simulink model "Torque_System_Identification"  (R2018a)
settings: Solver=FixedStepAuto  StartTime=0.0  StopTime=inf  FixedStep=.015  RelTol=1e-3  EnableMultiTasking=on
libraries: raspberrypilib x28, hdlsllib x25, simulink x15
(part 2 of 2)

== system Torque_System_Identification/Control System/Black Box/radio_steering read message (Master --> Slave) ==
  Inport : Inport
  Mux : Mux
      settings: DisplayOption=signals
  Read Bit Set : simulink/Logic and Bit Operations/Bit Set  iBit=7
      settings: SourceProductName=Simulink  SourceProductBaseCode=SL
  uint8_t 1 : Constant  OutDataTypeStr=uint8
  uint8_t 2 : Constant  OutDataTypeStr=uint8
  uint8_t 3 : Constant  OutDataTypeStr=uint8
  Out1 : Outport
  wires:
  Read Bit Set/1 -> Mux/1  "Addres/RW Byte radio_steering Teensy Status will be returned here"
  uint8_t 1/1 -> Mux/2  "Junk will be returned here"
  Inport/1 -> Read Bit Set/1
  uint8_t 3/1 -> Mux/4  "Byte 1 will be returned here"
  Mux/1 -> Out1/1
  uint8_t 2/1 -> Mux/3  "Byte 0 will be returned here"

== system Torque_System_Identification/Control System/Black Box/radio_steering return message (Slave --> Master) ==
  In1 : Inport
  8 bytes concatinated converted to double : DataTypeConversion  OutDataTypeStr=double  RndMeth=Nearest
  Bit Concat : hdlsllib/Logic and Bit Operations/Bit Concat  numInputs=2
      settings: SourceProductName=HDL Coder  SourceProductBaseCode=HD
  Bytes of the return message : Display
      settings: Format=decimal (Stored Integer)
  Data Type Conversion : DataTypeConversion  OutDataTypeStr=int16  RndMeth=Nearest
  Demux : Demux
  Display : Display
      settings: Format=binary (Stored Integer)
  Display1 : Display
      settings: Format=decimal (Stored Integer)
  Display2 : Display
      settings: Format=binary (Stored Integer)
  radio_steering : Outport
  wires:
  8 bytes concatinated converted to double/1 -> Display1/1, radio_steering/1  "radio_steering"
  Demux/2 -> Display2/1  "Slave Status"
  Demux/1 -> Display/1  "Previous Data"
  In1/1 -> Bytes of the return message/1, Demux/1
  Bit Concat/1 -> Data Type Conversion/1
  Demux/4 -> Bit Concat/1
  Demux/3 -> Bit Concat/2
  Data Type Conversion/1 -> 8 bytes concatinated converted to double/1

== system Torque_System_Identification/Control System/Black Box/radio_throttle read message (Master --> Slave) ==
  Inport : Inport
  Mux : Mux
      settings: DisplayOption=signals
  Read Bit Set : simulink/Logic and Bit Operations/Bit Set  iBit=7
      settings: SourceProductName=Simulink  SourceProductBaseCode=SL
  uint8_t 1 : Constant  OutDataTypeStr=uint8
  uint8_t 2 : Constant  OutDataTypeStr=uint8
  uint8_t 3 : Constant  OutDataTypeStr=uint8
  Out1 : Outport
  wires:
  Read Bit Set/1 -> Mux/1  "Addres/RW Byte radio_throttle Teensy Status will be returned here"
  uint8_t 1/1 -> Mux/2  "Junk will be returned here"
  Inport/1 -> Read Bit Set/1
  uint8_t 3/1 -> Mux/4  "Byte 1 will be returned here"
  Mux/1 -> Out1/1
  uint8_t 2/1 -> Mux/3  "Byte 0 will be returned here"

== system Torque_System_Identification/Control System/Black Box/radio_throttle return message (Slave --> Master) ==
  In1 : Inport
  8 bytes concatinated converted to double : DataTypeConversion  OutDataTypeStr=double  RndMeth=Nearest
  Bit Concat : hdlsllib/Logic and Bit Operations/Bit Concat  numInputs=2
      settings: SourceProductName=HDL Coder  SourceProductBaseCode=HD
  Bytes of the return message : Display
      settings: Format=decimal (Stored Integer)
  Data Type Conversion : DataTypeConversion  OutDataTypeStr=int16  RndMeth=Nearest
  Demux : Demux
  Display : Display
      settings: Format=binary (Stored Integer)
  Display1 : Display
      settings: Format=decimal (Stored Integer)
  Display2 : Display
      settings: Format=binary (Stored Integer)
  radio_throttle : Outport
  wires:
  8 bytes concatinated converted to double/1 -> Display1/1, radio_throttle/1  "radio_throttle"
  Demux/2 -> Display2/1  "Slave Status"
  Demux/1 -> Display/1  "Previous Data"
  In1/1 -> Bytes of the return message/1, Demux/1
  Bit Concat/1 -> Data Type Conversion/1
  Demux/4 -> Bit Concat/1
  Demux/3 -> Bit Concat/2
  Data Type Conversion/1 -> 8 bytes concatinated converted to double/1

== system Torque_System_Identification/Control System/Black Box/servo_out Write Message (Master --> Slave) ==
  In1 : Inport
  Bit Slice2 : hdlsllib/Logic and Bit Operations/Bit Slice  lidx=15  ridx=8
  Bit Slice3 : hdlsllib/Logic and Bit Operations/Bit Slice  lidx=7  ridx=0
  Display5 : Display
      settings: Format=decimal (Stored Integer)
  Mux : Mux  Inputs=2
      settings: DisplayOption=signals
  Out1 : Outport
  wires:
  In1/1 -> Display5/1, Bit Slice3/1, Bit Slice2/1  "Servo"
  Mux/1 -> Out1/1
  Bit Slice3/1 -> Mux/1
  Bit Slice2/1 -> Mux/2

== system Torque_System_Identification/Control System/Black Box/throttle_left_front Write Message (Master --> Slave) ==
  In1 : Inport
  Bit Slice : hdlsllib/Logic and Bit Operations/Bit Slice  lidx=15  ridx=8
  Bit Slice1 : hdlsllib/Logic and Bit Operations/Bit Slice  lidx=7  ridx=0
  Display4 : Display
  Mux : Mux  Inputs=2
      settings: DisplayOption=signals
  Output : Outport
  wires:
  Mux/1 -> Output/1
  Bit Slice/1 -> Display4/1, Mux/2
  Bit Slice1/1 -> Mux/1
  In1/1 -> Bit Slice/1, Bit Slice1/1

== system Torque_System_Identification/Control System/Black Box/throttle_left_rear Write Message (Master --> Slave) ==
  In1 : Inport
  Bit Slice : hdlsllib/Logic and Bit Operations/Bit Slice  lidx=15  ridx=8
  Bit Slice1 : hdlsllib/Logic and Bit Operations/Bit Slice  lidx=7  ridx=0
  Display4 : Display
  Mux : Mux  Inputs=2
      settings: DisplayOption=signals
  Output : Outport
  wires:
  In1/1 -> Bit Slice1/1, Bit Slice/1
  Bit Slice1/1 -> Mux/1
  Bit Slice/1 -> Mux/2, Display4/1
  Mux/1 -> Output/1

== system Torque_System_Identification/Control System/Black Box/throttle_right_front Write Message (Master --> Slave) ==
  In1 : Inport
  Bit Slice : hdlsllib/Logic and Bit Operations/Bit Slice  lidx=15  ridx=8
  Bit Slice1 : hdlsllib/Logic and Bit Operations/Bit Slice  lidx=7  ridx=0
  Display4 : Display
  Mux : Mux  Inputs=2
      settings: DisplayOption=signals
  Output : Outport
  wires:
  Mux/1 -> Output/1
  Bit Slice/1 -> Display4/1, Mux/2
  Bit Slice1/1 -> Mux/1
  In1/1 -> Bit Slice/1, Bit Slice1/1

== system Torque_System_Identification/Control System/Black Box/throttle_right_rear Write Message (Master --> Slave) ==
  In1 : Inport
  Bit Slice : hdlsllib/Logic and Bit Operations/Bit Slice  lidx=15  ridx=8
  Bit Slice1 : hdlsllib/Logic and Bit Operations/Bit Slice  lidx=7  ridx=0
  Display4 : Display
  Mux : Mux  Inputs=2
      settings: DisplayOption=signals
  Output : Outport
  wires:
  In1/1 -> Bit Slice1/1, Bit Slice/1
  Bit Slice1/1 -> Mux/1
  Bit Slice/1 -> Mux/2, Display4/1
  Mux/1 -> Output/1

== system Torque_System_Identification/Control System/Black Box/velocity_FL read message (Master --> Slave) ==
  Inport : Inport
  Mux : Mux
      settings: DisplayOption=signals
  Read Bit Set : simulink/Logic and Bit Operations/Bit Set  iBit=7
      settings: SourceProductName=Simulink  SourceProductBaseCode=SL
  uint8_t 1 : Constant  OutDataTypeStr=uint8
  uint8_t 2 : Constant  OutDataTypeStr=uint8
  uint8_t 3 : Constant  OutDataTypeStr=uint8
  Out1 : Outport
  wires:
  Read Bit Set/1 -> Mux/1  "Addres/RW Byte velocity_FL Teensy Status will be returned here"
  uint8_t 1/1 -> Mux/2  "Junk will be returned here"
  Inport/1 -> Read Bit Set/1
  uint8_t 3/1 -> Mux/4  "Byte 1 will be returned here"
  Mux/1 -> Out1/1
  uint8_t 2/1 -> Mux/3  "Byte 0 will be returned here"

== system Torque_System_Identification/Control System/Black Box/velocity_FL return message (Slave --> Master) ==
  In1 : Inport
  8 bytes concatinated converted to double : DataTypeConversion  OutDataTypeStr=double  RndMeth=Nearest
  Bit Concat : hdlsllib/Logic and Bit Operations/Bit Concat  numInputs=2
      settings: SourceProductName=HDL Coder  SourceProductBaseCode=HD
  Bytes of the return message : Display
      settings: Format=decimal (Stored Integer)
  Data Type Conversion : DataTypeConversion  OutDataTypeStr=int16  RndMeth=Nearest
  Demux : Demux
  Display : Display
      settings: Format=binary (Stored Integer)
  Display1 : Display
      settings: Format=decimal (Stored Integer)
  Display2 : Display
      settings: Format=binary (Stored Integer)
  velocity_FL : Outport
  wires:
  8 bytes concatinated converted to double/1 -> Display1/1, velocity_FL/1  "velocity_FL"
  Demux/2 -> Display2/1  "Slave Status"
  Demux/1 -> Display/1  "Previous Data"
  In1/1 -> Bytes of the return message/1, Demux/1
  Bit Concat/1 -> Data Type Conversion/1
  Demux/4 -> Bit Concat/1
  Demux/3 -> Bit Concat/2
  Data Type Conversion/1 -> 8 bytes concatinated converted to double/1

== system Torque_System_Identification/Control System/Black Box/velocity_FR read message (Master --> Slave) ==
  Inport : Inport
  Mux : Mux
      settings: DisplayOption=signals
  Read Bit Set : simulink/Logic and Bit Operations/Bit Set  iBit=7
      settings: SourceProductName=Simulink  SourceProductBaseCode=SL
  uint8_t 1 : Constant  OutDataTypeStr=uint8
  uint8_t 2 : Constant  OutDataTypeStr=uint8
  uint8_t 3 : Constant  OutDataTypeStr=uint8
  Out1 : Outport
  wires:
  Read Bit Set/1 -> Mux/1  "Addres/RW Byte velocity_FR Teensy Status will be returned here"
  uint8_t 1/1 -> Mux/2  "Junk will be returned here"
  Inport/1 -> Read Bit Set/1
  uint8_t 3/1 -> Mux/4  "Byte 1 will be returned here"
  Mux/1 -> Out1/1
  uint8_t 2/1 -> Mux/3  "Byte 0 will be returned here"

== system Torque_System_Identification/Control System/Black Box/velocity_FR return message (Slave --> Master) ==
  In1 : Inport
  8 bytes concatinated converted to double : DataTypeConversion  OutDataTypeStr=double  RndMeth=Nearest
  Bit Concat : hdlsllib/Logic and Bit Operations/Bit Concat  numInputs=2
      settings: SourceProductName=HDL Coder  SourceProductBaseCode=HD
  Bytes of the return message : Display
      settings: Format=decimal (Stored Integer)
  Data Type Conversion : DataTypeConversion  OutDataTypeStr=int16  RndMeth=Nearest
  Demux : Demux
  Display : Display
      settings: Format=binary (Stored Integer)
  Display1 : Display
      settings: Format=decimal (Stored Integer)
  Display2 : Display
      settings: Format=binary (Stored Integer)
  velocity_FR : Outport
  wires:
  8 bytes concatinated converted to double/1 -> Display1/1, velocity_FR/1  "radio_throttle"
  Demux/2 -> Display2/1  "Slave Status"
  Demux/1 -> Display/1  "Previous Data"
  In1/1 -> Bytes of the return message/1, Demux/1
  Bit Concat/1 -> Data Type Conversion/1
  Demux/4 -> Bit Concat/1
  Demux/3 -> Bit Concat/2
  Data Type Conversion/1 -> 8 bytes concatinated converted to double/1

== system Torque_System_Identification/Control System/Black Box/velocity_RL read message (Master --> Slave) ==
  Inport : Inport
  Mux : Mux
      settings: DisplayOption=signals
  Read Bit Set : simulink/Logic and Bit Operations/Bit Set  iBit=7
      settings: SourceProductName=Simulink  SourceProductBaseCode=SL
  uint8_t 1 : Constant  OutDataTypeStr=uint8
  uint8_t 2 : Constant  OutDataTypeStr=uint8
  uint8_t 3 : Constant  OutDataTypeStr=uint8
  Out1 : Outport
  wires:
  Read Bit Set/1 -> Mux/1  "Addres/RW Byte velocity_RL Teensy Status will be returned here"
  uint8_t 1/1 -> Mux/2  "Junk will be returned here"
  Inport/1 -> Read Bit Set/1
  uint8_t 3/1 -> Mux/4  "Byte 1 will be returned here"
  Mux/1 -> Out1/1
  uint8_t 2/1 -> Mux/3  "Byte 0 will be returned here"

== system Torque_System_Identification/Control System/Black Box/velocity_RL return message (Slave --> Master) ==
  In1 : Inport
  8 bytes concatinated converted to double : DataTypeConversion  OutDataTypeStr=double  RndMeth=Nearest
  Bit Concat : hdlsllib/Logic and Bit Operations/Bit Concat  numInputs=2
      settings: SourceProductName=HDL Coder  SourceProductBaseCode=HD
  Bytes of the return message : Display
      settings: Format=decimal (Stored Integer)
  Data Type Conversion : DataTypeConversion  OutDataTypeStr=int16  RndMeth=Nearest
  Demux : Demux
  Display : Display
      settings: Format=binary (Stored Integer)
  Display1 : Display
      settings: Format=decimal (Stored Integer)
  Display2 : Display
      settings: Format=binary (Stored Integer)
  velocity_RL : Outport
  wires:
  8 bytes concatinated converted to double/1 -> Display1/1, velocity_RL/1  "velocity_RL"
  Demux/2 -> Display2/1  "Slave Status"
  Demux/1 -> Display/1  "Previous Data"
  In1/1 -> Bytes of the return message/1, Demux/1
  Bit Concat/1 -> Data Type Conversion/1
  Demux/4 -> Bit Concat/1
  Demux/3 -> Bit Concat/2
  Data Type Conversion/1 -> 8 bytes concatinated converted to double/1

== system Torque_System_Identification/Control System/Black Box/velocity_RR read message (Master --> Slave) ==
  Inport : Inport
  Mux : Mux
      settings: DisplayOption=signals
  Read Bit Set : simulink/Logic and Bit Operations/Bit Set  iBit=7
      settings: SourceProductName=Simulink  SourceProductBaseCode=SL
  uint8_t 1 : Constant  OutDataTypeStr=uint8
  uint8_t 2 : Constant  OutDataTypeStr=uint8
  uint8_t 3 : Constant  OutDataTypeStr=uint8
  Out1 : Outport
  wires:
  Read Bit Set/1 -> Mux/1  "Addres/RW Byte velocity_RR Teensy Status will be returned here"
  uint8_t 1/1 -> Mux/2  "Junk will be returned here"
  Inport/1 -> Read Bit Set/1
  uint8_t 3/1 -> Mux/4  "Byte 1 will be returned here"
  Mux/1 -> Out1/1
  uint8_t 2/1 -> Mux/3  "Byte 0 will be returned here"

== system Torque_System_Identification/Control System/Black Box/velocity_RR return message (Slave --> Master) ==
  In1 : Inport
  8 bytes concatinated converted to double : DataTypeConversion  OutDataTypeStr=double  RndMeth=Nearest
  Bit Concat : hdlsllib/Logic and Bit Operations/Bit Concat  numInputs=2
      settings: SourceProductName=HDL Coder  SourceProductBaseCode=HD
  Bytes of the return message : Display
      settings: Format=decimal (Stored Integer)
  Data Type Conversion : DataTypeConversion  OutDataTypeStr=int16  RndMeth=Nearest
  Demux : Demux
  Display : Display
      settings: Format=binary (Stored Integer)
  Display1 : Display
      settings: Format=decimal (Stored Integer)
  Display2 : Display
      settings: Format=binary (Stored Integer)
  velocity_RR : Outport
  wires:
  8 bytes concatinated converted to double/1 -> Display1/1, velocity_RR/1  "velocity_RR"
  Demux/2 -> Display2/1  "Slave Status"
  Demux/1 -> Display/1  "Previous Data"
  In1/1 -> Bytes of the return message/1, Demux/1
  Bit Concat/1 -> Data Type Conversion/1
  Demux/4 -> Bit Concat/1
  Demux/3 -> Bit Concat/2
  Data Type Conversion/1 -> 8 bytes concatinated converted to double/1
